simulink model "district_model"  (R2026a)
settings: Solver=VariableStepAuto  StopTime=p.sim_stop
PostLoadFcn:
  | dm_dir = fileparts(get_param(bdroot, 'FileName'));
  | if ~contains(path, dm_dir), addpath(dm_dir); end, clear dm_dir
  | if ~exist('p', 'var') || ~isstruct(p) || ~isfield(p, 'n_edge_devices')
  |     [p, PatientBus] = district_model_params();
  | elseif ~exist('PatientBus', 'var')
  |     [~, PatientBus] = district_model_params();
  | end
InitFcn:
  | district_model_check(bdroot);
values from neighbouring files (symbols this model uses):
  m = [mdl '/']    [build_district_model.m]    (also in run_district_model.m)
undefined symbols (not defined in the file or in its folder): n
Description:
  | District DR screening: group arrivals, capture, AI quality check (good / borderline / bad), restoration, AI grading, and doctor review. Variables: district_model_params.m. Built by build_district_model.m.
settings Model: Creator=yashc  LastModifiedBy=yashc

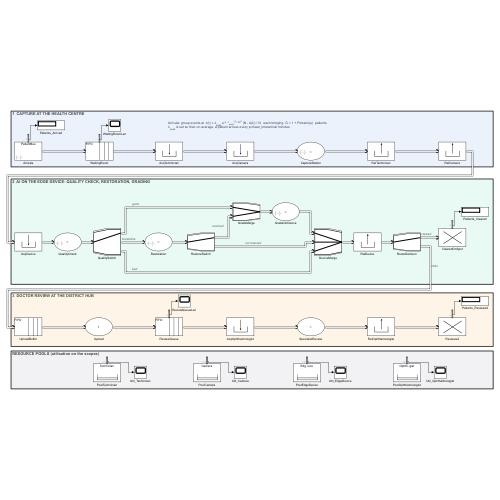
[thumbnail: Simulink's stored preview of the top-level diagram]
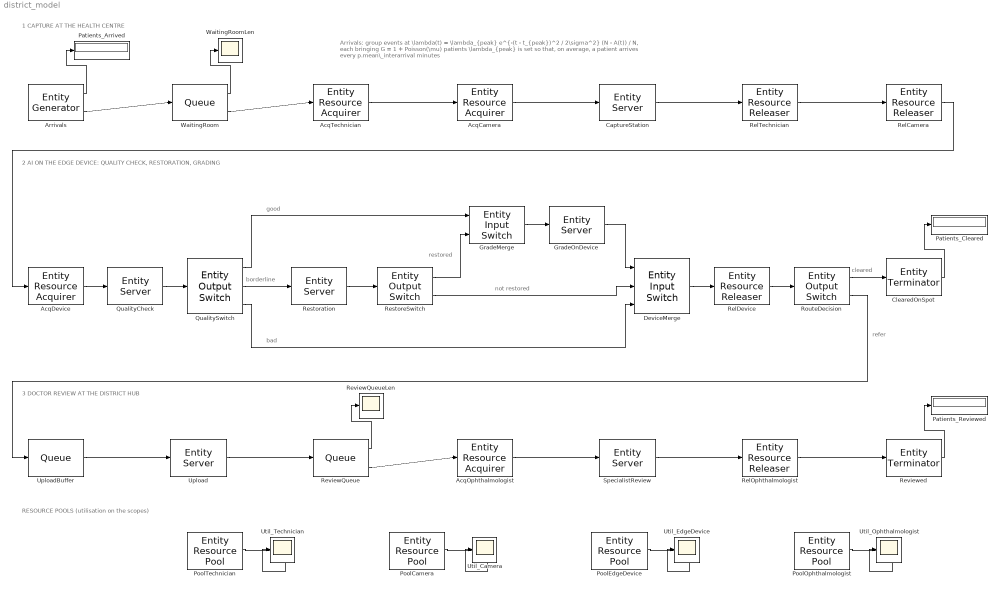
== system district_model ==
  note: 1 CAPTURE AT THE HEALTH CENTRE
  note: 2 AI ON THE EDGE DEVICE: QUALITY CHECK, RESTORATION, GRADING
  note: 3 DOCTOR REVIEW AT THE DISTRICT HUB
  note: RESOURCE POOLS (utilisation on the scopes)
  note: Arrivals: group events at  \lambda(t) = \lambda_{peak} e^{-(t - t_{peak})^2 / 2\sigma^2} (N - A(t)) / N,  each bringing  G = 1 + Poisson(\mu)  patients
      | \lambda_{peak} is set so that, on average, a patient arrives every p.mean\_interarrival minutes
  note: good
  note: borderline
  note: bad
  note: restored
  note: not restored
  note: cleared
  note: refer
  AcqCamera : EntityResourceAcquirer  InputPortMessageModes=m  OutputPortMessageModes=m  NumberWaitingEntities=p.n_technicians  ResourceName=Camera
      settings: OutputPortMap=o3
  AcqDevice : EntityResourceAcquirer  InputPortMessageModes=m  OutputPortMessageModes=m  NumberWaitingEntities=p.cap_waiting_room  ResourceName=EdgeDevice
      settings: OutputPortMap=o3
  AcqOphthalmologist : EntityResourceAcquirer  InputPortMessageModes=m  OutputPortMessageModes=m  ResourceName=Ophthalmologist
      settings: OutputPortMap=o3
  AcqTechnician : EntityResourceAcquirer  InputPortMessageModes=m  OutputPortMessageModes=m  ResourceName=Technician
      settings: OutputPortMap=o3
  Arrivals : EntityGenerator  OutputPortMessageModes=n,m  TimeSource=MATLAB action  IntergenerationTimeAction=|  GenerateEntityAtSimulationStart=off  GenerateAction=|  NumberEntitiesDeparted=on  EntityType=Bus object  EntityTypeName=PatientBus
      IntergenerationTimeAction=|
      | % Group arrivals: events at rate
      | %   lambda(t) = lambda_peak * exp(-(t - t_peak)^2 / (2 sigma^2)) * (N - A(t)) / N
      | % (A(t): patients so far), each bringing G = 1 + Poisson(mu) patients.
      | % Drawn by thinning: candidates at lambda_peak, each kept with
      | % probability lambda(t) / lambda_peak.
      | persistent seeded tclock remaining arrived lam
      | if isempty(seeded)
      |     rng(p.seed * 100 + 1, 'twister'); seeded = 1;
      |     tclock = 0; remaining = 0; arrived = 0;
      |     lam = district_peak_rate(p);          % one patient every p.mean_interarrival min, on average
      | end
      | if remaining > 0
      |     % the rest of a group arrives at the same moment
      |     remaining = remaining - 1;
      |     arrived = arrived + 1;
      |     dt = 0;
      | else
      |     tc = tclock;
      |     dt = 1e9;                             % no more arrivals this session
      |     while arrived < p.N && tc < p.sim_stop
      |         tc = tc - log(rand) / lam;        % a candidate at the peak rate
      |         rate = lam * exp(-(tc - p.t_peak)^2 / (2 * p.sigma^2)) * (p.N - arrived) / p.N;
      |         if rand * lam <= rate
      |             k = 0; L = exp(-p.mu); u = rand;   % group size - 1 ~ Poisson(mu)
      |             while u > L
      |                 k = k + 1; u = u * rand;
      |             end
      |             remaining = min(k, p.N - arrived - 1);
      |             arrived = arrived + 1;
      |             dt = tc - tclock;
      |             break
      |         end
      |     end
      | end
      | tclock = tclock + dt;
      GenerateAction=|
      | persistent seeded
      | if isempty(seeded), rng(p.seed * 100 + 2, 'twister'); seeded = 1; end
      | entity.true_status   = double(rand < p.prevalence_referable);
      | entity.quality_class = 0;
      | entity.restored      = 0;
      | entity.ungradable    = 0;
      | entity.attempts      = 0;
      | entity.flagged       = 0;
      | entity.route         = 1;
      settings: OutputPortMap=o0,o3
  CaptureStation : EntityServer  InputPortMessageModes=m  OutputPortMessageModes=m  Capacity=Inf  ServiceTimeValue=p.t_capture  ServiceCompleteAction=entity.attempts = entity.attempts + 1;
  ClearedOnSpot : EntityTerminator  InputPortMessageModes=m  NumberEntitiesArrived=on
      settings: OutputPortMap=o0
  DeviceMerge : EntityInputSwitch  InputPortMessageModes=m,m,m  OutputPortMessageModes=m  NumberInputPorts=3
      settings: InputPortMap=u1,u2,u3
  GradeMerge : EntityInputSwitch  InputPortMessageModes=m,m  OutputPortMessageModes=m
  GradeOnDevice : EntityServer  InputPortMessageModes=m  OutputPortMessageModes=m  Capacity=Inf  ServiceTimeValue=p.t_grade  ServiceCompleteAction=|
      | % the AI grades a gradeable image
      | persistent seeded
      | if isempty(seeded), rng(p.seed * 100 + 5, 'twister'); seeded = 1; end
      | if entity.true_status == 1
      |     entity.flagged = double(rand < p.sensitivity);
      | else
      |     entity.flagged = double(rand > p.specificity);
      | end
      | entity.route = entity.flagged + 1;       % 1 cleared on the spot, 2 to the doctor
  Patients_Arrived : Display
  Patients_Cleared : Display
  Patients_Reviewed : Display
  PoolCamera : EntityResourcePool  ResourceName=Camera  ResourceAmount=p.n_cameras  AverageUtilization=on
      settings: OutputPortMap=o1
  PoolEdgeDevice : EntityResourcePool  ResourceName=EdgeDevice  ResourceAmount=p.n_edge_devices  AverageUtilization=on
      settings: OutputPortMap=o1
  PoolOphthalmologist : EntityResourcePool  ResourceName=Ophthalmologist  ResourceAmount=p.n_ophthalmologists  AverageUtilization=on
      settings: OutputPortMap=o1
  PoolTechnician : EntityResourcePool  ResourceName=Technician  ResourceAmount=p.n_technicians  AverageUtilization=on
      settings: OutputPortMap=o1
  QualityCheck : EntityServer  InputPortMessageModes=m  OutputPortMessageModes=m  Capacity=Inf  ServiceTimeValue=p.t_quality  ServiceCompleteAction=|
      | % the AI sorts the image: 1 good, 2 borderline, 3 bad
      | persistent seeded
      | if isempty(seeded), rng(p.seed * 100 + 3, 'twister'); seeded = 1; end
      | r = rand * (p.p_pass + p.p_repair + p.p_reject);
      | if r < p.p_pass
      |     entity.quality_class = 1;
      | elseif r < p.p_pass + p.p_repair
      |     entity.quality_class = 2;
      | else
      |     entity.quality_class = 3;
      |     % another capture if the gate is in and captures remain,
      |     % otherwise to the doctor ungraded
      |     if p.include_gate && entity.attempts < p.max_attempts
      |         entity.route = 3;
      |     else
      |         entity.ungradable = 1; entity.flagged = 1; entity.route = 2;
      |     end
      | end
  QualitySwitch : EntityOutputSwitch  InputPortMessageModes=m  OutputPortMessageModes=m,m,m  NumberOutputPorts=3  SwitchingCriterion=From attribute  SwitchAttributeName=quality_class
      settings: OutputPortMap=o0,o1,o2
  RelCamera : EntityResourceReleaser  InputPortMessageModes=m  OutputPortMessageModes=m  ResourceName=Camera
  RelDevice : EntityResourceReleaser  InputPortMessageModes=m  OutputPortMessageModes=m  ResourceName=EdgeDevice
  RelOphthalmologist : EntityResourceReleaser  InputPortMessageModes=m  OutputPortMessageModes=m  ResourceName=Ophthalmologist
  RelTechnician : EntityResourceReleaser  InputPortMessageModes=m  OutputPortMessageModes=m  ResourceName=Technician
  Restoration : EntityServer  InputPortMessageModes=m  OutputPortMessageModes=m  Capacity=Inf  ServiceTimeValue=p.t_restore  ServiceCompleteAction=|
      | % restoration saves p_restore of borderline images
      | persistent seeded
      | if isempty(seeded), rng(p.seed * 100 + 4, 'twister'); seeded = 1; end
      | if rand < p.p_restore
      |     entity.restored = 1;
      | else
      |     entity.restored = 2;
      |     % another capture if the gate is in and captures remain,
      |     % otherwise to the doctor ungraded
      |     if p.include_gate && entity.attempts < p.max_attempts
      |         entity.route = 3;
      |     else
      |         entity.ungradable = 1; entity.flagged = 1; entity.route = 2;
      |     end
      | end
  RestoreSwitch : EntityOutputSwitch  InputPortMessageModes=m  OutputPortMessageModes=m,m  SwitchingCriterion=From attribute  SwitchAttributeName=restored
  ReviewQueue : Queue  InputPortMessageModes=m  OutputPortMessageModes=n,m  Capacity=p.cap_review_queue  NumberEntitiesInBlock=on
      settings: OutputPortMap=o1,o5
  ReviewQueueLen : Scope
  Reviewed : EntityTerminator  InputPortMessageModes=m  NumberEntitiesArrived=on
      settings: OutputPortMap=o0
  RouteDecision : EntityOutputSwitch  InputPortMessageModes=m  OutputPortMessageModes=m,m  SwitchingCriterion=From attribute  SwitchAttributeName=route
  SpecialistReview : EntityServer  InputPortMessageModes=m  OutputPortMessageModes=m  Capacity=Inf  ServiceTimeValue=p.t_review
  Upload : EntityServer  InputPortMessageModes=m  OutputPortMessageModes=m  Capacity=1  ServiceTimeValue=p.t_upload
  UploadBuffer : Queue  InputPortMessageModes=m  OutputPortMessageModes=m  Capacity=p.cap_upload_buffer
  Util_Camera : Scope
  Util_EdgeDevice : Scope
  Util_Ophthalmologist : Scope
  Util_Technician : Scope
  WaitingRoom : Queue  InputPortMessageModes=m  OutputPortMessageModes=n,m  Capacity=p.cap_waiting_room  NumberEntitiesInBlock=on
      settings: OutputPortMap=o1,o5
  WaitingRoomLen : Scope
  wires:
  Arrivals/2 -> WaitingRoom/1
  WaitingRoom/2 -> AcqTechnician/1
  AcqTechnician/1 -> AcqCamera/1
  AcqCamera/1 -> CaptureStation/1
  CaptureStation/1 -> RelTechnician/1
  RelTechnician/1 -> RelCamera/1
  RelCamera/1 -> AcqDevice/1
  AcqDevice/1 -> QualityCheck/1
  QualityCheck/1 -> QualitySwitch/1
  QualitySwitch/1 -> GradeMerge/1
  QualitySwitch/2 -> Restoration/1
  QualitySwitch/3 -> DeviceMerge/3
  Restoration/1 -> RestoreSwitch/1
  RestoreSwitch/1 -> GradeMerge/2
  RestoreSwitch/2 -> DeviceMerge/2
  GradeMerge/1 -> GradeOnDevice/1
  GradeOnDevice/1 -> DeviceMerge/1
  DeviceMerge/1 -> RelDevice/1
  RelDevice/1 -> RouteDecision/1
  RouteDecision/1 -> ClearedOnSpot/1
  RouteDecision/2 -> UploadBuffer/1
  UploadBuffer/1 -> Upload/1
  Upload/1 -> ReviewQueue/1
  ReviewQueue/2 -> AcqOphthalmologist/1
  AcqOphthalmologist/1 -> SpecialistReview/1
  SpecialistReview/1 -> RelOphthalmologist/1
  RelOphthalmologist/1 -> Reviewed/1
  Arrivals/1 -> Patients_Arrived/1
  WaitingRoom/1 -> WaitingRoomLen/1
  ClearedOnSpot/1 -> Patients_Cleared/1
  ReviewQueue/1 -> ReviewQueueLen/1
  Reviewed/1 -> Patients_Reviewed/1
  PoolTechnician/1 -> Util_Technician/1
  PoolCamera/1 -> Util_Camera/1
  PoolEdgeDevice/1 -> Util_EdgeDevice/1
  PoolOphthalmologist/1 -> Util_Ophthalmologist/1
